simulink model "asbCubeSatACS"  (R2023b)
settings: Solver=FixedStepAuto  StartTime=0.0  StopTime=10.0  FixedStep=CubeSatTimeStep  RelTol=1e-3  EnableMultiTasking=on
libraries: aerolibutil x5, matrix_library x5, aerolibsatdyn x2, sharedtransform x2, simulink_extras x1, slpidlib x1
settings Model: DataDictionary=asbCubeSatModelData.sldd  SnapshotInterval=1  Creator=The MathWorks, Inc.  LastModifiedBy=Adin Sacho-Tanzer
settings SolverCC: ZeroCrossControl=DisableAll  AlgebraicLoopSolver=TrustRegion  MaxZcPerStep=1
settings DataIOCC: LimitDataPoints=on  SaveFormat=Array  SaveOutput=off  DSMLogging=off  SaveTime=off  ReturnWorkspaceOutputs=off
settings OptimizationCC: DefaultParameterBehavior=Inlined  OptimizeBlockIOStorage=off  BufferReuse=off  GlobalBufferReuse=off  ExpressionFolding=off  ExpressionDepthLimit=2147483647  LocalBlockOutputs=off  InitFltsAndDblsToZero=on  LifeSpan=inf  OptimizeDataStoreBuffers=off  BusAssignmentInplaceUpdate=off
settings DebuggingCC: ArtificialAlgebraicLoopMsg=none  SolverPrmCheckMsg=warning  FcnCallInpInsideContextMsg=warning  UnconnectedInputMsg=warning  UnconnectedOutputMsg=warning  UnconnectedLineMsg=warning  StateNameClashWarn=warning  PregeneratedLibrarySubsystemCodeDiagnostic=none  SFUnexpectedBacktrackingDiag=warning  SFNoUnconditionalDefaultTransitionDiag=warning  SFExecutionAtInitializationDiag=none  ArithmeticOperatorsInVariantConditions=warning
settings HardwareCC: ProdBitPerPointer=32  ProdBitPerSizeT=32  ProdBitPerPtrDiffT=32  ProdLargestAtomicFloat=None  ProdIntDivRoundTo=Undefined  ProdEndianess=Unspecified  ProdWordSize=32  ProdHWDeviceType=32-bit Generic
settings ModelReferenceCC: EnableRefExpFcnMdlSchedulingChecks=on  PropagateSignalLabelsOutOfModel=off
settings SFSimCC: SimUseLocalCustomCode=off
settings RTWCC: RTWUseLocalCustomCode=off  DLArmComputeVersion=19.05
settings CodeAppCC: StateflowObjectComments=on
settings GRTTargetCC: TargetFcnLib=ansi_tfl_tmw.mat  TargetLangStandard=C89/C90 (ANSI)  CombineOutputUpdateFcns=off  MatFileLogging=off  GRTInterface=on
settings ConfigComp: CovMetricSettings=dw  CovSaveCumulativeToWorkspaceVar=on  CovSaveSingleToWorkspaceVar=on  CovExternalEMLEnable=off

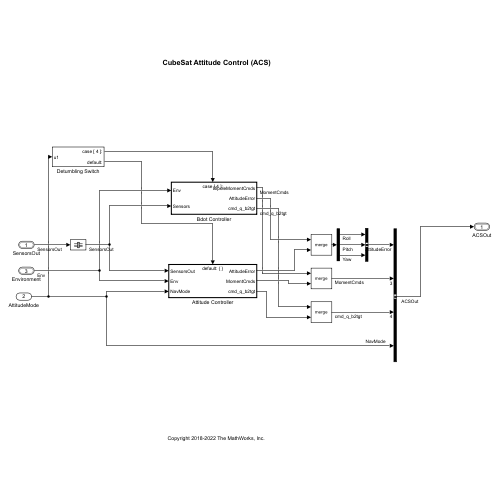
[thumbnail: Simulink's stored preview of the top-level diagram]
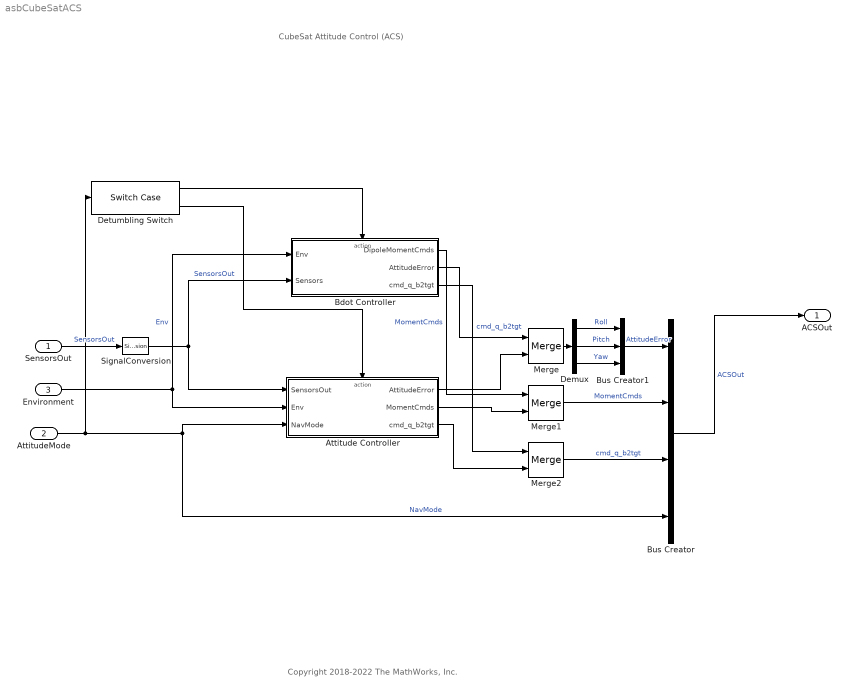
== system asbCubeSatACS ==
  note: Copyright 2018-2022 The MathWorks, Inc.
  note: CubeSat Attitude Control (ACS)
  SensorsOut : Inport  OutDataTypeStr=Bus: StatesOutBus
  AttitudeMode : Inport  Port=2  OutDataTypeStr=double  PortDimensions=1
  Environment : Inport  Port=3  OutDataTypeStr=Bus: EnvBus  PortDimensions=1
  Attitude Controller : Subsystem
  Bdot Controller : Subsystem
  Bus Creator : BusCreator  Inputs=4  OutDataTypeStr=Bus: ACSOutBus  NonVirtualBus=on
  Bus Creator1 : BusCreator  Inputs=3  OutDataTypeStr=Bus: AttitudeErrorBus
  Demux : Demux  Outputs=3
  Detumbling Switch : SwitchCase  CaseConditions={4}
  Merge : Merge
  Merge1 : Merge
  Merge2 : Merge
  SignalConversion : SignalConversion  ConversionOutput=Virtual bus  OverrideOpt=off
  ACSOut : Outport  OutDataTypeStr=Bus: ACSOutBus  PortDimensions=1  VectorParamsAs1DForOutWhenUnconnected=off  BusOutputAsStruct=on
  wires:
  SensorsOut/1 -> SignalConversion/1  "SensorsOut"
  Bus Creator/1 -> ACSOut/1  "ACSOut"
  Environment/1 -> Attitude Controller/2(Env), Bdot Controller/1(Env)  "Env"
  SignalConversion/1 -> Attitude Controller/1(SensorsOut), Bdot Controller/2(Sensors)  "SensorsOut"
  Detumbling Switch/1 -> Bdot Controller/Action
  Detumbling Switch/2 -> Attitude Controller/Action
  AttitudeMode/1 -> Detumbling Switch/1, Bus Creator/4, Attitude Controller/3(NavMode)  "NavMode"
  Attitude Controller/1(AttitudeError) -> Merge/2
  Attitude Controller/2(MomentCmds) -> Merge1/2
  Attitude Controller/3(cmd_q_b2tgt) -> Merge2/2
  Merge2/1 -> Bus Creator/3  "cmd_q_b2tgt"
  Merge1/1 -> Bus Creator/2  "MomentCmds"
  Bdot Controller/3(cmd_q_b2tgt) -> Merge2/1  "cmd_q_b2tgt"
  Bdot Controller/2(AttitudeError) -> Merge/1
  Bdot Controller/1(DipoleMomentCmds) -> Merge1/1  "MomentCmds"
  Merge/1 -> Demux/1
  Demux/2 -> Bus Creator1/2  "Pitch"
  Demux/1 -> Bus Creator1/1  "Roll"
  Bus Creator1/1 -> Bus Creator/1  "AttitudeError"
  Demux/3 -> Bus Creator1/3  "Yaw"

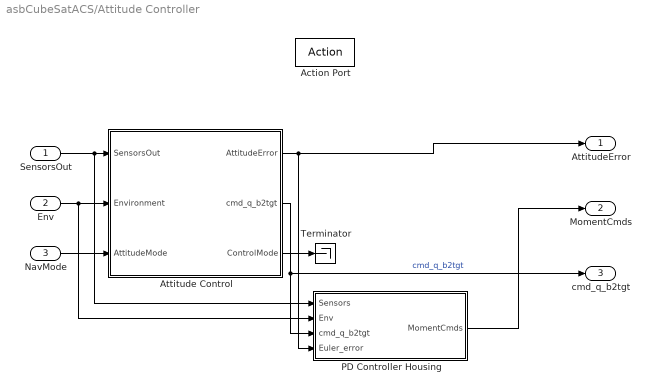
== system asbCubeSatACS/Attitude Controller ==
  SensorsOut : Inport
  Env : Inport  Port=2
  NavMode : Inport  Port=3
  Action Port : ActionPort  ActionPortLabel=default:
  Attitude Control : Subsystem
  PD Controller Housing : Subsystem
  Terminator : Terminator
  AttitudeError : Outport
  MomentCmds : Outport  Port=2
  cmd_q_b2tgt : Outport  Port=3
  wires:
  Attitude Control/1(AttitudeError) -> PD Controller Housing/4(Euler_error), AttitudeError/1
  Attitude Control/3(" ControlMode") -> Terminator/1
  Attitude Control/2(cmd_q_b2tgt) -> PD Controller Housing/3(cmd_q_b2tgt), cmd_q_b2tgt/1  "cmd_q_b2tgt"
  NavMode/1 -> Attitude Control/3("AttitudeMode ")
  Env/1 -> PD Controller Housing/2(Env), Attitude Control/2(Environment)
  SensorsOut/1 -> PD Controller Housing/1(Sensors), Attitude Control/1("SensorsOut ")
  PD Controller Housing/1(MomentCmds) -> MomentCmds/1

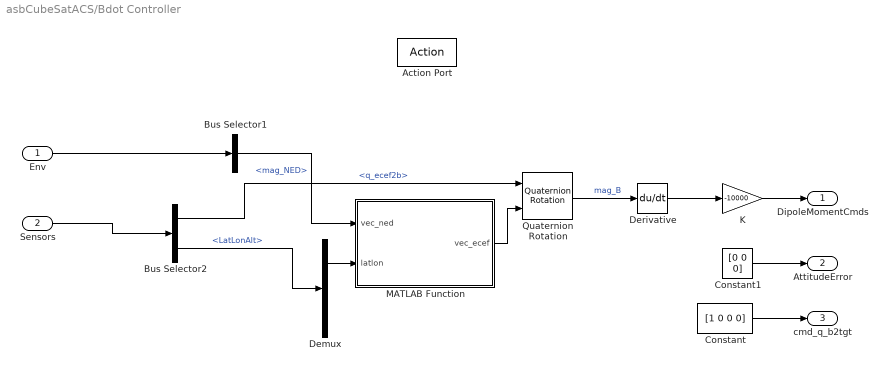
== system asbCubeSatACS/Bdot Controller ==
  Env : Inport
  Sensors : Inport  Port=2
  Action Port : ActionPort  ActionPortLabel=case [ 4 ]:
  Bus Selector1 : BusSelector  OutputSignals=mag_NED
  Bus Selector2 : BusSelector  OutputSignals=q_ecef2b,LatLonAlt
  Constant : Constant  Value=[1 0 0 0]
  Constant1 : Constant  Value=[0 0 0]
  Demux : Demux  Outputs=[2 1]
  Derivative : Derivative
  K : Gain  Gain=-10000
  MATLAB Function : MATLAB Function  TreatAsAtomicUnit=on
  Quaternion Rotation : aerolibutil/Quaternion Rotation
  DipoleMomentCmds : Outport
  AttitudeError : Outport  Port=2
  cmd_q_b2tgt : Outport  Port=3
  wires:
  Derivative/1 -> K/1
  MATLAB Function/1(vec_ecef) -> Quaternion Rotation/2
  Bus Selector2/1 -> Quaternion Rotation/1  "<q_ecef2b>"
  Env/1 -> Bus Selector1/1
  K/1 -> DipoleMomentCmds/1
  Bus Selector1/1 -> MATLAB Function/1(vec_ned)  "<mag_NED>"
  Quaternion Rotation/1 -> Derivative/1  "mag_B"
  Demux/1 -> MATLAB Function/2(latlon)
  Bus Selector2/2 -> Demux/1  "<LatLonAlt>"
  Sensors/1 -> Bus Selector2/1
  Constant/1 -> cmd_q_b2tgt/1
  Constant1/1 -> AttitudeError/1

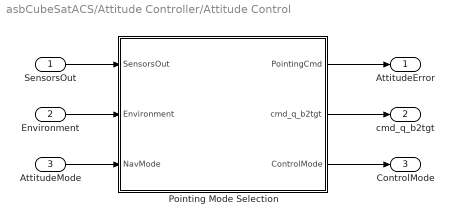
== system asbCubeSatACS/Attitude Controller/Attitude Control ==
  "SensorsOut " : Inport  OutDataTypeStr=Bus: StatesOutBus
  Environment : Inport  Port=2
  "AttitudeMode " : Inport  Port=3
  Pointing Mode Selection : Stateflow chart  RequirementInfo="{}  %GIDa_a065c7c8_537d_4123_b3cc_6e7e7008a32c"  TreatAsAtomicUnit=on
  AttitudeError : Outport  VectorParamsAs1DForOutWhenUnconnected=off
  cmd_q_b2tgt : Outport  Port=2  VectorParamsAs1DForOutWhenUnconnected=off
  " ControlMode" : Outport  Port=3  VectorParamsAs1DForOutWhenUnconnected=off
  wires:
  "SensorsOut "/1 -> Pointing Mode Selection/1(SensorsOut)
  Pointing Mode Selection/3(ControlMode) -> " ControlMode"/1
  "AttitudeMode "/1 -> Pointing Mode Selection/3(NavMode)
  Environment/1 -> Pointing Mode Selection/2(Environment)
  Pointing Mode Selection/1(PointingCmd) -> AttitudeError/1
  Pointing Mode Selection/2(cmd_q_b2tgt) -> cmd_q_b2tgt/1

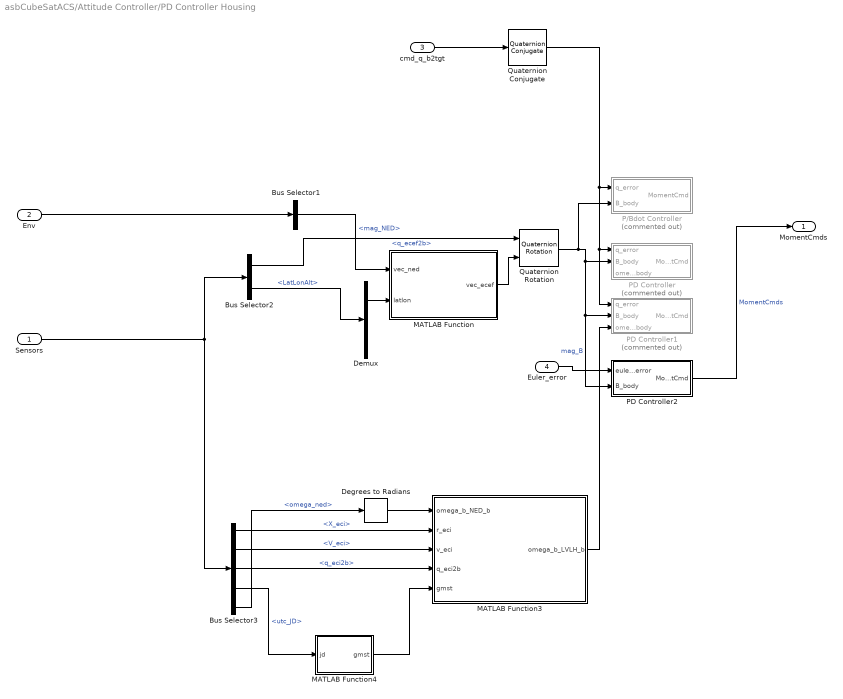
== system asbCubeSatACS/Attitude Controller/PD Controller Housing ==
  Sensors : Inport
  Env : Inport  Port=2
  cmd_q_b2tgt : Inport  Port=3
  Euler_error : Inport  Port=4
  Bus Selector1 : BusSelector  OutputSignals=mag_NED
  Bus Selector2 : BusSelector  OutputSignals=q_ecef2b,LatLonAlt
  Bus Selector3 : BusSelector  OutputSignals=X_eci,V_eci,q_eci2b,utc_JD,omega_ned
  Degrees to Radians : simulink_extras/Transformations/Degrees to Radians
  Demux : Demux  Outputs=[2 1]
  MATLAB Function : MATLAB Function  TreatAsAtomicUnit=on
  MATLAB Function3 : MATLAB Function  TreatAsAtomicUnit=on
  MATLAB Function4 : MATLAB Function  TreatAsAtomicUnit=on
  P/Bdot Controller : Subsystem  Commented=on
  PD Controller : Subsystem  Commented=on
  PD Controller1 : Subsystem  Commented=on
  PD Controller2 : Subsystem
  Quaternion Conjugate : aerolibutil/Quaternion Conjugate
  Quaternion Rotation : aerolibutil/Quaternion Rotation
  MomentCmds : Outport
  wires:
  Bus Selector1/1 -> MATLAB Function/1(vec_ned)  "<mag_NED>"
  Demux/1 -> MATLAB Function/2(latlon)
  Bus Selector2/1 -> Quaternion Rotation/1  "<q_ecef2b>"
  MATLAB Function/1(vec_ecef) -> Quaternion Rotation/2
  Env/1 -> Bus Selector1/1
  Sensors/1 -> Bus Selector2/1, Bus Selector3/1
  Quaternion Rotation/1 -> P/Bdot Controller/2(B_body), PD Controller2/2(B_body), PD Controller1/2(B_body), PD Controller/2(B_body)  "mag_B"
  Bus Selector2/2 -> Demux/1  "<LatLonAlt>"
  cmd_q_b2tgt/1 -> Quaternion Conjugate/1
  Quaternion Conjugate/1 -> P/Bdot Controller/1(q_error), PD Controller1/1(q_error), PD Controller/1(q_error)
  Bus Selector3/4 -> MATLAB Function4/1(jd)  "<utc_JD>"
  MATLAB Function4/1(gmst) -> MATLAB Function3/5(gmst)
  Bus Selector3/3 -> MATLAB Function3/4(q_eci2b)  "<q_eci2b>"
  Bus Selector3/2 -> MATLAB Function3/3(v_eci)  "<V_eci>"
  Bus Selector3/1 -> MATLAB Function3/2(r_eci)  "<X_eci>"
  Bus Selector3/5 -> Degrees to Radians/1  "<omega_ned>"
  MATLAB Function3/1(omega_b_LVLH_b) -> PD Controller1/3(omega_body)
  Degrees to Radians/1 -> MATLAB Function3/1(omega_b_NED_b)
  Euler_error/1 -> PD Controller2/1(euler_error)
  PD Controller2/1(MomentCmd) -> MomentCmds/1  "MomentCmds"

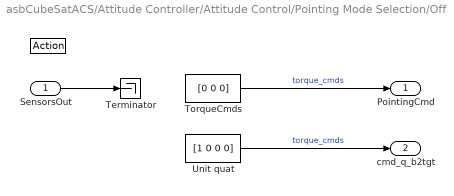
== system asbCubeSatACS/Attitude Controller/Attitude Control/Pointing Mode Selection/Off ==
  SensorsOut : Inport  OutDataTypeStr=Bus: StatesOutBus
  " " : ActionPort
      settings: CopyFcn=Stateflow.SLINSF.SimulinkMan.removeBlockPreDeleteFcn  PreDeleteFcn=Stateflow.SLINSF.SimulinkMan.unsafePredeleteFcn
  Terminator : Terminator
  TorqueCmds : Constant  Value=[0 0 0]
  Unit quat : Constant  Value=[1 0 0 0]
  PointingCmd : Outport  RequirementInfo="{}  %GIDa_4dc055f9_6cac_42e1_8ddb_4145586b89f5"  VectorParamsAs1DForOutWhenUnconnected=off
  cmd_q_b2tgt : Outport  RequirementInfo="{}  %GIDa_ca05d0a6_a581_4c3e_b3a0_cd281b586de8"  Port=2  VectorParamsAs1DForOutWhenUnconnected=off
  wires:
  SensorsOut/1 -> Terminator/1
  TorqueCmds/1 -> PointingCmd/1  "torque_cmds"
  Unit quat/1 -> cmd_q_b2tgt/1  "torque_cmds"

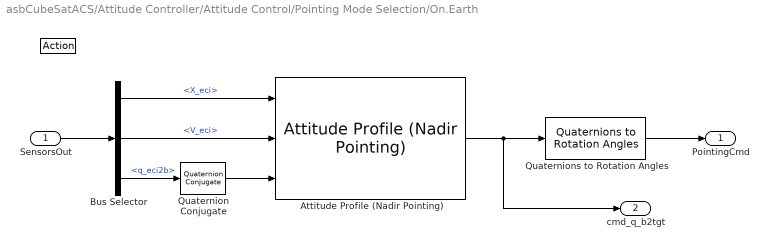
== system asbCubeSatACS/Attitude Controller/Attitude Control/Pointing Mode Selection/On.Earth ==
  SensorsOut : Inport  OutDataTypeStr=Bus: StatesOutBus
  " " : ActionPort
      settings: CopyFcn=Stateflow.SLINSF.SimulinkMan.removeBlockPreDeleteFcn  PreDeleteFcn=Stateflow.SLINSF.SimulinkMan.unsafePredeleteFcn
  Attitude Profile (Nadir Pointing) : aerolibsatdyn/Attitude Profile (Nadir Pointing)  outputError=on  outputFinalAttitude=off  portFrame=ICRF  pointingMode=Point at nadir  celestialTarget=Sun  tunablePointing=off  primaryAlignmentSrc=Dialog  primaryAlignment=[0 0 1]  secondaryAlignmentSrc=Dialog  secondaryAlignment=[1 0 0]  constraintFrame=LVLH  primaryConstraintSrc=Dialog  primaryConstraint=[1 0 0]  secondaryConstraintSrc=Dialog  secondaryConstraint=[0 1 0]
  Bus Selector : BusSelector  OutputSignals=X_eci,V_eci,q_eci2b
  Quaternion Conjugate : aerolibutil/Quaternion Conjugate
  Quaternions to Rotation Angles : sharedtransform/Quaternions to Rotation Angles  rotationOrder=XYZ  aMode=aMode
  PointingCmd : Outport  VectorParamsAs1DForOutWhenUnconnected=off
  cmd_q_b2tgt : Outport  RequirementInfo="{}  %GIDa_69a01501_0b6a_41cf_b570_f5b49bb229cd"  Port=2  VectorParamsAs1DForOutWhenUnconnected=off
  wires:
  Quaternions to Rotation Angles/1 -> PointingCmd/1
  Bus Selector/3 -> Quaternion Conjugate/1  "<q_eci2b>"
  Bus Selector/2 -> Attitude Profile (Nadir Pointing)/2  "<V_eci>"
  SensorsOut/1 -> Bus Selector/1
  Bus Selector/1 -> Attitude Profile (Nadir Pointing)/1  "<X_eci>"
  Quaternion Conjugate/1 -> Attitude Profile (Nadir Pointing)/3
  Attitude Profile (Nadir Pointing)/1 -> cmd_q_b2tgt/1, Quaternions to Rotation Angles/1

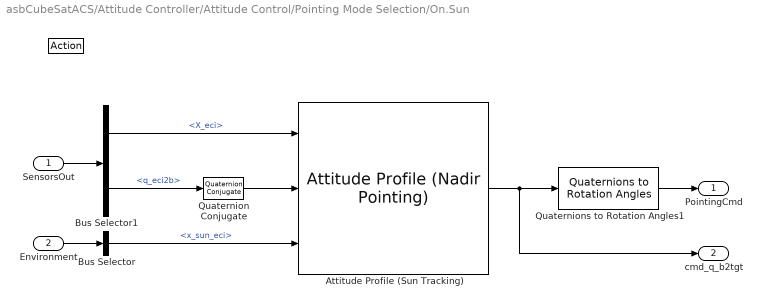
== system asbCubeSatACS/Attitude Controller/Attitude Control/Pointing Mode Selection/On.Sun ==
  SensorsOut : Inport  OutDataTypeStr=Bus: StatesOutBus
  Environment : Inport  Port=2  OutDataTypeStr=Bus: EnvBus
  " " : ActionPort
      settings: CopyFcn=Stateflow.SLINSF.SimulinkMan.removeBlockPreDeleteFcn  PreDeleteFcn=Stateflow.SLINSF.SimulinkMan.unsafePredeleteFcn
  Attitude Profile (Sun Tracking) : aerolibsatdyn/Attitude Profile (Nadir Pointing)  outputError=on  outputFinalAttitude=off  portFrame=ICRF  pointingMode=Custom  celestialTarget=Sun  tunablePointing=off  primaryAlignmentSrc=Dialog  primaryAlignment=[0 0 -1]  secondaryAlignmentSrc=Dialog  secondaryAlignment=[1 0 0]  constraintFrame=ICRF  primaryConstraintSrc=Port  primaryConstraint=[1 0 0]  secondaryConstraintSrc=Dialog  secondaryConstraint=[0 0 1]
  Bus Selector : BusSelector  OutputSignals=x_sun_eci
  Bus Selector1 : BusSelector  OutputSignals=X_eci,q_eci2b
  Quaternion Conjugate : aerolibutil/Quaternion Conjugate
  Quaternions to Rotation Angles1 : sharedtransform/Quaternions to Rotation Angles  rotationOrder=XYZ  aMode=aMode
  PointingCmd : Outport  VectorParamsAs1DForOutWhenUnconnected=off
  cmd_q_b2tgt : Outport  Port=2  VectorParamsAs1DForOutWhenUnconnected=off
  wires:
  Attitude Profile (Sun Tracking)/1 -> Quaternions to Rotation Angles1/1, cmd_q_b2tgt/1
  SensorsOut/1 -> Bus Selector1/1
  Environment/1 -> Bus Selector/1
  Quaternions to Rotation Angles1/1 -> PointingCmd/1
  Bus Selector/1 -> Attitude Profile (Sun Tracking)/3  "<x_sun_eci>"
  Quaternion Conjugate/1 -> Attitude Profile (Sun Tracking)/2
  Bus Selector1/2 -> Quaternion Conjugate/1  "<q_eci2b>"
  Bus Selector1/1 -> Attitude Profile (Sun Tracking)/1  "<X_eci>"

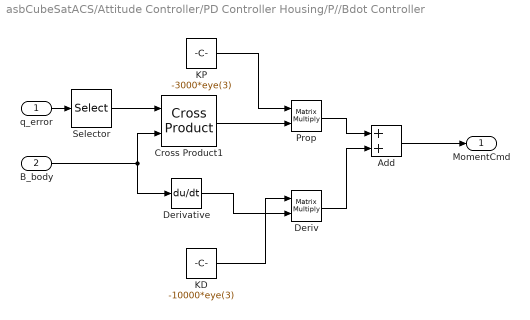
== system asbCubeSatACS/Attitude Controller/PD Controller Housing/P//Bdot Controller ==
  q_error : Inport
  B_body : Inport  Port=2
  Add : Sum
  Cross Product1 : matrix_library/Cross Product
  Deriv : Product  Multiplication=Matrix(*)
  Derivative : Derivative
  KD : Constant  Value=-10000*eye(3)
  KP : Constant  Value=-3000*eye(3)  VectorParams1D=off
  Prop : Product  Multiplication=Matrix(*)
  Selector : Selector  InputPortWidth=4  IndexOptions=Index vector (dialog)  Indices=[2 3 4]  OutputSizes=1
  MomentCmd : Outport
  wires:
  B_body/1 -> Cross Product1/2, Derivative/1
  KD/1 -> Deriv/1
  KP/1 -> Prop/1
  Cross Product1/1 -> Prop/2
  Prop/1 -> Add/1
  Deriv/1 -> Add/2
  Add/1 -> MomentCmd/1
  q_error/1 -> Selector/1
  Selector/1 -> Cross Product1/1
  Derivative/1 -> Deriv/2

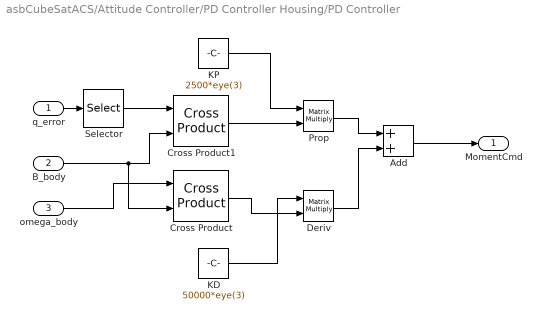
== system asbCubeSatACS/Attitude Controller/PD Controller Housing/PD Controller ==
  q_error : Inport
  B_body : Inport  Port=2
  omega_body : Inport  Port=3
  Add : Sum
  Cross Product : matrix_library/Cross Product
  Cross Product1 : matrix_library/Cross Product
  Deriv : Product  Multiplication=Matrix(*)
  KD : Constant  Value=50000*eye(3)
  KP : Constant  Value=2500*eye(3)  VectorParams1D=off
  Prop : Product  Multiplication=Matrix(*)
  Selector : Selector  InputPortWidth=4  IndexOptions=Index vector (dialog)  Indices=[2 3 4]  OutputSizes=1
  MomentCmd : Outport
  wires:
  omega_body/1 -> Cross Product/1
  B_body/1 -> Cross Product1/2, Cross Product/2
  KD/1 -> Deriv/1
  Cross Product/1 -> Deriv/2
  KP/1 -> Prop/1
  Cross Product1/1 -> Prop/2
  Prop/1 -> Add/1
  Deriv/1 -> Add/2
  Add/1 -> MomentCmd/1
  q_error/1 -> Selector/1
  Selector/1 -> Cross Product1/1

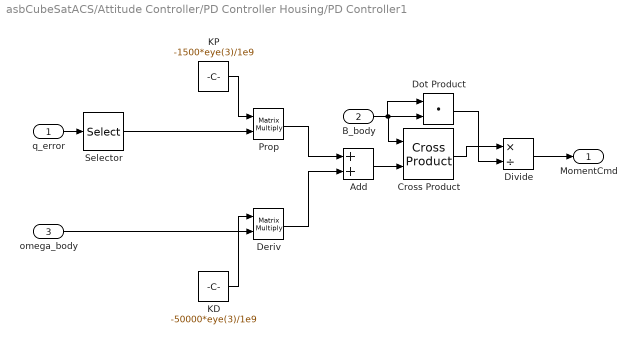
== system asbCubeSatACS/Attitude Controller/PD Controller Housing/PD Controller1 ==
  q_error : Inport
  B_body : Inport  Port=2
  omega_body : Inport  Port=3
  Add : Sum
  Cross Product : matrix_library/Cross Product
  Deriv : Product  Multiplication=Matrix(*)
  Divide : Product  Inputs=*/
  Dot Product : DotProduct  OutDataTypeStr=Inherit: Inherit via internal rule
  KD : Constant  Value=-50000*eye(3)/1e9
  KP : Constant  Value=-1500*eye(3)/1e9  VectorParams1D=off
  Prop : Product  Multiplication=Matrix(*)
  Selector : Selector  InputPortWidth=4  IndexOptions=Index vector (dialog)  Indices=[2 3 4]  OutputSizes=1
  MomentCmd : Outport
  wires:
  KD/1 -> Deriv/1
  omega_body/1 -> Deriv/2
  KP/1 -> Prop/1
  Selector/1 -> Prop/2
  Prop/1 -> Add/1
  Deriv/1 -> Add/2
  q_error/1 -> Selector/1
  Add/1 -> Cross Product/2
  B_body/1 -> Dot Product/2, Cross Product/1, Dot Product/1
  Dot Product/1 -> Divide/2
  Cross Product/1 -> Divide/1
  Divide/1 -> MomentCmd/1

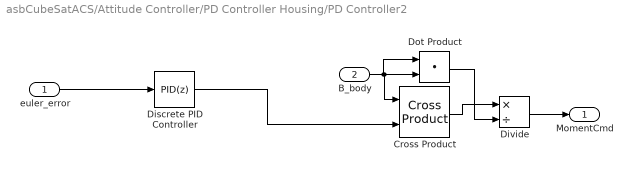
== system asbCubeSatACS/Attitude Controller/PD Controller Housing/PD Controller2 ==
  euler_error : Inport
  B_body : Inport  Port=2
  Cross Product : matrix_library/Cross Product
  Discrete PID Controller : slpidlib/PID Controller  Controller=PID  Form=Parallel  TimeDomain=Discrete-time  UseExternalTs=off  SampleTime=-1  IntegratorMethod=Forward Euler  FilterMethod=Forward Euler  ControllerParametersSource=internal  P=5e-05/1e4  I=0  UseKiTs=off  D=0.017/1e4  N=100  UseFilter=off  TunerSelectOption=Transfer Function Based (PID Tuner App)  InitialConditionSource=internal  InitialConditionForIntegrator=0  InitialConditionForFilter=0  DifferentiatorICPrevScaledInput=0  ExternalReset=none  TrackingMode=off  Kt=1  LimitOutput=off  SatLimitsSource=internal  UpperSaturationLimit=inf  LowerSaturationLimit=-inf  LinearizeAsGain=off  AntiWindupMode=none  Kb=1  LimitIntegrator=off  UpperIntegratorSaturationLimit=inf  LowerIntegratorSaturationLimit=-inf  POutMin=[]  POutMax=[]  IOutMin=[]  IOutMax=[]  DOutMin=[]  DOutMax=[]  NOutMin=[]  NOutMax=[]  SumOutMin=[]  SumOutMax=[]  SaturationOutMin=[]  SaturationOutMax=[]  PParamMin=[]  PParamMax=[]  IParamMin=[]  IParamMax=[]  DParamMin=[]  DParamMax=[]  NParamMin=[]  NParamMax=[]  KbParamMin=[]  KbParamMax=[]  KtParamMin=[]  KtParamMax=[]  KbOutMin=[]  KbOutMax=[]  KtOutMin=[]  KtOutMax=[]  IntegratorOutMin=[]  IntegratorOutMax=[]  FilterOutMin=[]  FilterOutMax=[]  SumI1OutMin=[]  SumI1OutMax=[]  SumI2OutMin=[]  SumI2OutMax=[]  SumI3OutMin=[]  SumI3OutMax=[]  SumI4OutMin=[]  SumI4OutMax=[]  SumDOutMin=[]  SumDOutMax=[]  DifferentiatorOutMin=[]  DifferentiatorOutMax=[]  FilterDiffOutCoefMin=[]  FilterDiffOutCoefMax=[]  ReciprocalOutMin=[]  ReciprocalOutMax=[]  SumDenOutMin=[]  SumDenOutMax=[]  SumNumOutMin=[]  SumNumOutMax=[]  DivideOutMin=[]  DivideOutMax=[]  UdiffTsProdOutMin=[]  UdiffTsProdOutMax=[]  NTsProdOutMin=[]  NTsProdOutMax=[]  UintegralTsProdOutMin=[]  UintegralTsProdOutMax=[]  UngainTsProdOutMin=[]  UngainTsProdOutMax=[]  ClampingZeroOutDataTypeStr=Inherit: Inherit via back propagation  ClampingZeroOutMin=[]  ClampingZeroOutMax=[]  FilterDenConstantOutDataTypeStr=Inherit: Inherit via back propagation  FilterDenConstantOutMin=[]  FilterDenConstantOutMax=[]  PCopyOutDataTypeStr=Inherit: Inherit via back propagation  PCopyOutMin=[]  PCopyOutMax=[]  NCopyOutDataTypeStr=Inherit: Inherit via back propagation  NCopyOutMin=[]  NCopyOutMax=[]  IntegratorContinuousStateAttributes=''  IntegratorStateMustResolveToSignalObject=off  IntegratorRTWStateStorageClass=Auto  FilterContinuousStateAttributes=''  FilterStateMustResolveToSignalObject=off  FilterRTWStateStorageClass=Auto  ParallelPVariant=InternalParameters  IdealPVariant=Disabled  IVariant=InternalParameters  DVariant=InternalParameters  IntegratorVariant=Discrete  SatVariant=Disabled  AWVariant=Passthrough  PCopyVariant=Disabled  TRVariant=Disabled  FdbkBlocksVariant=Forward  IdealPFdbkVariant=Disabled  SatFdbkVariant=Disabled  DerivativeFilterVariant=Differentiator  NVariant=Passthrough  NCopyVariant=Disabled_SignalSpec  FilterICVariant=InternalICsDifferentiator  IntegratorICVariant=InternalICs  ExternalResetVariant=Disabled  TRSumVariant=Passthrough  SumFdbkVariant=Disabled  SumVariant=Sum_PID  TsampFilterVariant=InternalTs  TsampNgainVariant=Passthrough  TsampIntegralVariant=Disabled_SignalSpec  ExternalSaturationOutDataTypeStr=Inherit: Same as second input
      settings: LibrarySourceBlock=simulink/Discrete/Discrete PID Controller
  Divide : Product  Inputs=*/
  Dot Product : DotProduct  OutDataTypeStr=Inherit: Inherit via internal rule
  MomentCmd : Outport
  wires:
  euler_error/1 -> Discrete PID Controller/1
  Discrete PID Controller/1 -> Cross Product/2
  B_body/1 -> Dot Product/2, Cross Product/1, Dot Product/1
  Dot Product/1 -> Divide/2
  Cross Product/1 -> Divide/1
  Divide/1 -> MomentCmd/1

== matlab function asbCubeSatACS/Attitude Controller/PD Controller Housing/MATLAB Function ==
  data: vec_ned input; vec_ecef output double size=[3 1]; latlon input
function vec_ecef = convert_ned2ecef(vec_ned, latlon)

vec_ecef = zeros(3,1);

uN = vec_ned(1);
vE = vec_ned(2);
wD = vec_ned(3);

lat = deg2rad(latlon(1));
lon = deg2rad(latlon(2));

sLat = sin(lat);
cLat = cos(lat);
sLon = sin(lon);
cLon = cos(lon);

vec_ecef(1) = -sLat*cLon*uN - sLon*vE - cLat*cLon*wD;
vec_ecef(2) = -sLat*sLon*uN + cLon*vE - cLat*sLon*wD;
vec_ecef(3) =  cLat*uN              - sLat*wD;

end

== matlab function asbCubeSatACS/Attitude Controller/PD Controller Housing/MATLAB Function3 ==
  data: omega_b_NED_b input; omega_b_LVLH_b output; r_eci input; v_eci input; q_eci2b input; gmst input
function omega_b_LVLH_b = fcn(omega_b_NED_b, r_eci, v_eci, q_eci2b, gmst)
%#codegen
% -----------------------------------------------------------------------
% Simulink MATLAB Function Block
% Convert omega_body/NED (body frame) -> omega_body/LVLH (body frame)
%
% INPUTS
%   omega_b_NED_b [3x1]  body angular velocity w.r.t. NED, in body (rad/s)
%   r_eci         [3x1]  ECI position (m)
%   v_eci         [3x1]  ECI velocity (m/s)
%   q_eci2b       [4x1]  quaternion ECI->body, SCALAR-FIRST [qs; qx; qy; qz]
%   gmst          [1x1]  Greenwich Mean Sidereal Time (rad)
%
% OUTPUT
%   omega_b_LVLH_b [3x1] body angular velocity w.r.t. LVLH, in body (rad/s)
%
% LVLH CONVENTION (RSW)
%   x = radial outward,  y = along-track,  z = cross-track ( -h )
%
% QUATERNION CONVENTION
%   Scalar-first: q = [qs; qx; qy; qz]
%   Rotation sense: v_body = C_b_ECI * v_eci
%   (matches MATLAB Aerospace Toolbox / Simulink default)
%
% EARTH MODEL
%   Spherical Earth for lat/lon from ECI position.
%   Replace with WGS-84 if higher fidelity is needed.
% -----------------------------------------------------------------------
 
    %% constants
    w_e = 7.2921159e-5;   % Earth rotation rate (rad/s)
    Re  = 6378137.0;      % Earth equatorial radius (m)
 
    %% 1  quaternion -> DCM  (ECI to body)
    qs = q_eci2b(1);  qx = q_eci2b(2);
    qy = q_eci2b(3);  qz = q_eci2b(4);
 
    C_b_ECI = ...
      [qs*qs+qx*qx-qy*qy-qz*qz,  2*(qx*qy+qs*qz),          2*(qx*qz-qs*qy);
       2*(qx*qy-qs*qz),          qs*qs-qx*qx+qy*qy-qz*qz,  2*(qy*qz+qs*qx);
       2*(qx*qz+qs*qy),          2*(qy*qz-qs*qx),          qs*qs-qx*qx-qy*qy+qz*qz];
 
    %% 2  LVLH frame  (from r, v in ECI)
    r_mag = norm(r_eci);
    r_hat = r_eci / r_mag;
 
    h_vec = cross(r_eci, v_eci);
    h_mag = norm(h_vec);
    h_hat = h_vec / h_mag;
 
    x_L = r_hat;                       % radial out
    z_L = -h_hat;                      % cross-track  (completes RHS)
    y_L = cross(z_L, x_L);            % along-track
 
    C_LVLH_ECI = [x_L';  y_L';  z_L'];
 
    %% 3  omega_LVLH/ECI  (in LVLH)
    omega_orb = h_mag / r_mag^2;       % instantaneous orbital rate
    omega_LVLH_ECI_lvlh = [0; 0; -omega_orb];
 
    %% 4  ECI -> ECEF rotation
    cg = cos(gmst);  sg = sin(gmst);
    C_ECEF_ECI = [ cg, sg, 0;
                  -sg, cg, 0;
                    0,  0, 1];
 
    %% 5  geodetic lat / lon  (spherical Earth)
    r_ecef = C_ECEF_ECI * r_eci;
    lon = atan2(r_ecef(2), r_ecef(1));
    lat = atan2(r_ecef(3), sqrt(r_ecef(1)^2 + r_ecef(2)^2));
 
    slat = sin(lat);  clat = cos(lat);
    slon = sin(lon);  clon = cos(lon);
 
    %% 6  DCM: ECEF -> NED
    C_NED_ECEF = [-slat*clon, -slat*slon,  clat;
                  -slon,       clon,        0;
                  -clat*clon, -clat*slon,  -slat];
 
    %% 7  DCM: ECI -> NED
    C_NED_ECI = C_NED_ECEF * C_ECEF_ECI;
 
    %% 8  velocity relative to ECEF, expressed in NED
    %      v_rel = v_eci - omega_earth x r  (both in ECI, then rotate)
    omega_e_eci = [0; 0; w_e];
    v_rel_eci   = v_eci - cross(omega_e_eci, r_eci);
    v_rel_ecef  = C_ECEF_ECI * v_rel_eci;
    v_ned       = C_NED_ECEF * v_rel_ecef;
 
    v_N = v_ned(1);
    v_E = v_ned(2);
 
    %% 9  omega_NED/ECI in NED
    %      transport rate  +  Earth rate
    Rh = r_mag;   % spherical: R + h = |r|
    omega_NED_ECI_ned = [ v_E / Rh  + w_e * clat;
                         -v_N / Rh;
                         -v_E * tan(lat) / Rh - w_e * slat];
 
    %% 10  omega_NED/LVLH in NED
    C_NED_LVLH          = C_NED_ECI * C_LVLH_ECI';
    omega_LVLH_ECI_ned  = C_NED_LVLH * omega_LVLH_ECI_lvlh;
    omega_NED_LVLH_ned  = omega_NED_ECI_ned - omega_LVLH_ECI_ned;
 
    %% 11  rotate correction into body and add
    C_b_NED        = C_b_ECI * C_NED_ECI';
    omega_b_LVLH_b = omega_b_NED_b + C_b_NED * omega_NED_LVLH_ned;
 
end

== matlab function asbCubeSatACS/Attitude Controller/PD Controller Housing/MATLAB Function4 ==
  data: jd input; gmst output
function gmst = jd2gmst(jd)
%JD2GMST Compute Greenwich Mean Sidereal Time from Julian Date.
%
%   Input:
%       jd   - Julian Date (UTC)
%
%   Output:
%       gmst - GMST in radians [0, 2*pi)
 
%#codegen
 
T_ut1 = (jd - 2451545.0) / 36525.0;
 
gmst_sec = 67310.54841 ...
         + (876600*3600 + 8640184.812866) * T_ut1 ...
         + 0.093104 * T_ut1^2 ...
         - 6.2e-6 * T_ut1^3;
 
gmst = mod(gmst_sec * (pi/43200), 2*pi);
 
end

== stateflow chart asbCubeSatACS/Attitude Controller/Attitude Control/Pointing Mode Selection ==
  state On
    state Transition
    state Earth
    state Sun
    (default) -> Transition
    Transition -> Sun [order 2] : [NavMode == 2]
        | {ControlMode = 2;}
    Sun -> Transition : [NavMode == 1]
        | {ControlMode = 1;}
    Transition -> Earth [order 1] : [NavMode == 1]
        | {ControlMode = 2;}
    Earth -> Transition : [NavMode == 2]
        | {ControlMode = 1;}
  state Off
  (default) -> Off
  Off -> On : [NavMode ~= 0]
      | {ControlMode = 1;}
  On -> Off : [NavMode == 0]
      | {ControlMode = 0;}
  data: sf_internal_action_state_placeholder_data local double size=1 =0; sf_internal_action_state_placeholder_data local double size=1 =0; sf_internal_action_state_placeholder_data local double size=1 =0; SensorsOut input Bus: StatesOutBus; Environment input; NavMode input; PointingCmd output =[0 0 0]'; cmd_q_b2tgt output; ControlMode output

== matlab function asbCubeSatACS/Bdot Controller/MATLAB Function ==
  data: vec_ned input; vec_ecef output double size=[3 1]; latlon input
function vec_ecef = convert_ned2ecef(vec_ned, latlon)

vec_ecef = zeros(3,1);

uN = vec_ned(1);
vE = vec_ned(2);
wD = vec_ned(3);

lat = deg2rad(latlon(1));
lon = deg2rad(latlon(2));

sLat = sin(lat);
cLat = cos(lat);
sLon = sin(lon);
cLon = cos(lon);

vec_ecef(1) = -sLat*cLon*uN - sLon*vE - cLat*cLon*wD;
vec_ecef(2) = -sLat*sLon*uN + cLon*vE - cLat*sLon*wD;
vec_ecef(3) =  cLat*uN              - sLat*wD;

end
